simulink model "ExtKalmanTracking"  (Simulink 7.5)
settings: Solver=ode45  StartTime=0.0  StopTime=20  FixedStep=0.01  MaxStep=0.01  RelTol=1e-3
libraries: simulink x1, simulink_extras x1
settings Model: Creator=Phil Goddard  LastModifiedBy=Phil Goddard

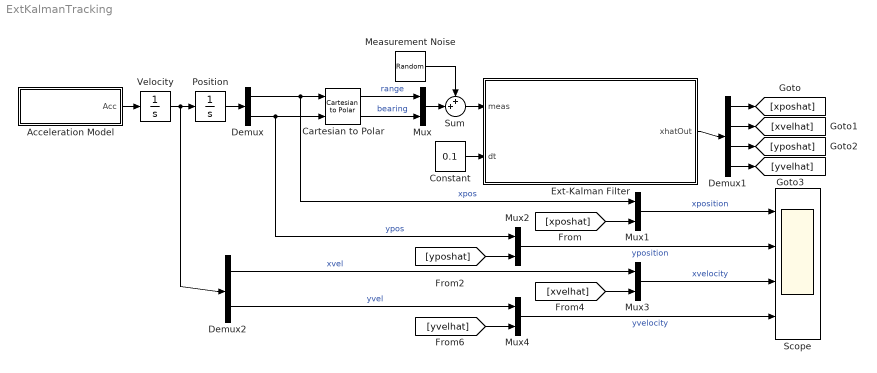
== system ExtKalmanTracking ==
  Acceleration Model : Subsystem
  Cartesian to Polar : simulink_extras/Transformations/Cartesian to Polar  SystemSampleTime=-1
  Constant : Constant  Value=0.1  OutDataType=fixdt(1, 16)  OutScaling=2^0
  Demux : Demux  Outputs=2
  Demux1 : Demux
  Demux2 : Demux  Outputs=2
  Ext-Kalman Filter : Stateflow chart  TreatAsAtomicUnit=on  SystemSampleTime=0.1
  Measurement Noise : RandomNumber  Variance=[50;0.005]  SampleTime=0.1
  Mux{,1..4} (5 alike) : Mux  Inputs=2
  Position : Integrator  InitialCondition=[-1000;1000]
  Scope : Scope  NumInputPorts=4
      settings: TimeRange=20  YMin=-1000~970~90~-2  YMax=1000~1030~110~2
  Sum : Sum  Inputs=++|  OutDataType=fixdt(1, 16)  OutScaling=2^0
  Velocity : Integrator  InitialCondition=[100;0]
  wires:
  Acceleration Model/1(Acc) -> Velocity/1
  Velocity/1 -> Position/1, Demux2/1
  Position/1 -> Demux/1
  Demux/1 -> Cartesian to Polar/1, Mux1/1  "xpos"
  Demux/2 -> Cartesian to Polar/2, Mux2/1  "ypos"
  Cartesian to Polar/1 -> Mux/1  "range"
  Cartesian to Polar/2 -> Mux/2  "bearing"
  Sum/1 -> Ext-Kalman Filter/1(meas)
  Ext-Kalman Filter/1(xhatOut) -> Demux1/1
  Demux1/1 -> [xposhat]
  Demux1/2 -> [xvelhat]
  Demux1/3 -> [yposhat]
  Demux1/4 -> [yvelhat]
  Mux1/1 -> Scope/1  "xposition"
  [xposhat] -> Mux1/2
  [yposhat] -> Mux2/2
  Mux2/1 -> Scope/2  "yposition"
  [xvelhat] -> Mux3/2
  Demux2/1 -> Mux3/1  "xvel"
  Mux3/1 -> Scope/3  "xvelocity"
  [yvelhat] -> Mux4/2
  Demux2/2 -> Mux4/1  "yvel"
  Mux4/1 -> Scope/4  "yvelocity"
  Mux/1 -> Sum/2
  Measurement Noise/1 -> Sum/1
  Constant/1 -> Ext-Kalman Filter/2(dt)

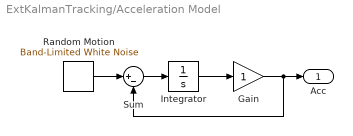
== system ExtKalmanTracking/Acceleration Model ==
  Gain : Gain  ParameterDataType=fixdt(1, 16)  ParameterScaling=2^0  OutDataType=fixdt(1, 16)  OutScaling=2^0
  Integrator : Integrator
  Random Motion : simulink/Sources/Band-Limited White Noise  SystemSampleTime=-1  Cov=[10;1]  Ts=0.01  seed=[23341]
  Sum : Sum  Inputs=|+-  OutDataType=fixdt(1, 16)  OutScaling=2^0
  Acc : Outport
  wires:
  Sum/1 -> Integrator/1
  Integrator/1 -> Gain/1
  Gain/1 -> Sum/2, Acc/1
  Random Motion/1 -> Sum/1

== matlab function Ext-Kalman Filter ==
  data: xhatOut output double; meas input double; dt input double
function xhatOut = ExtKalman(meas, dt)
% This Embedded MATLAB Function implements an extended Kalman filter used
% for object tracking.
%
% The states of the process are given by
% x = [x_position; x_velocity; y_position; y_velocity];
%
% and the measurements are given by
% y = [range; bearing]
%
% where 
% range = sqrt(x_position^2 + y_position^2)
% bearing = atan2(y_position/x_position)

% Author: Phil Goddard (phil@goddardconsulting.ca)
% Date: Q2, 2011.

% Define storage for the variables that need to persist
% between time periods.
persistent P xhat Q R
if isempty(P)
    % First time through the code so do some initialization
    xhat = [-900;80;950;20];
    P = zeros(4,4);
    Q =  diag([0 .1 0 .1]);
    R =  diag([50^2 0.005^2]);
end
% Calculate the Jacobians for the state and measurement equations
F = [1 dt 0 0;0 1 0 0;0 0 1 dt;0 0 0 1];
rangeHat = sqrt(xhat(1)^2+xhat(3)^2);
bearingHat = atan2(xhat(3),xhat(1));
yhat = [rangeHat; bearingHat]; 
H = [cos(bearingHat) 0 sin(bearingHat) 0;
    -sin(bearingHat)/rangeHat 0 cos(bearingHat)/rangeHat 0];

% Propogate the state and covariance matrices
xhat = F*xhat;
P = F*P*F' + Q;

% Calculate the Kalman gain
K = P*H'/(H*P*H' + R);

% Calculate the measurement residual
resid = meas - yhat;

% Update the state and covariance estimates
xhat = xhat + K*resid;
P = (eye(size(K,1))-K*H)*P;

% Post the results
xhatOut = xhat;
